simulink model "Context_Diagram"  (R2024a)
settings: Solver=VariableStepAuto  StartTime=0.0  StopTime=10.0  RelTol=1e-3
settings Model: Creator=kmara  LastModifiedBy=chico

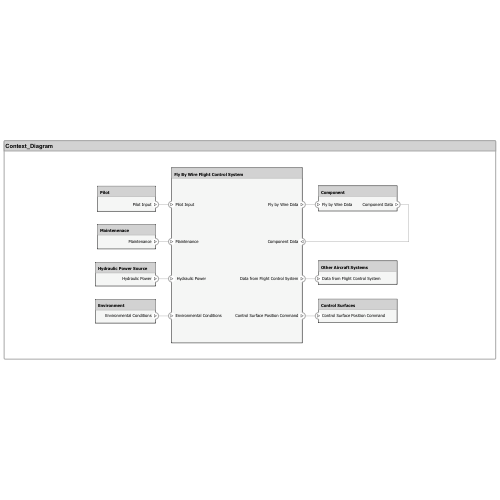
[thumbnail: Simulink's stored preview of the top-level diagram]
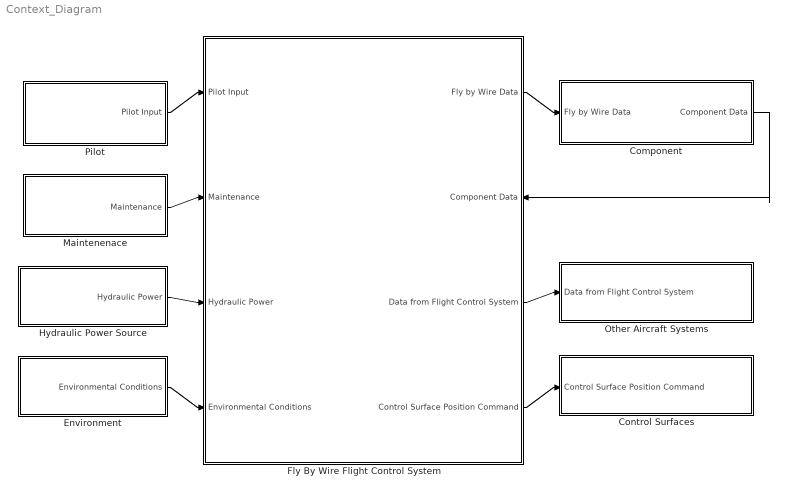
== system Context_Diagram ==
  Component : Subsystem
      settings: PortSchema="{\"entries\":[{\"content\":{\"headerSize\":26,\"margin\":15,\"minimumSpacing\":25,\"sides\":[{\"content\":{\"connectorIds\":[\"In1\"]},\"type\":\"ConnectorPlacement.EquallySpacedRectSide\",\"uuid\":\"b623a921-0a01-4933-aa95-d281e4fd472d\"},{\"content\":{\"connectorIds\":[\"Out1\"],\"side\":\"RIGHT\"},\"type\":\"ConnectorPlacement.EquallySpacedRectSide\",\"uuid\":\"7949cc00-59a5-498d-8900-6268840cf223\"},{\"content\":{\"side\":\"TOP\"},\"type\":\"ConnectorPlacement.EquallySpacedRectSide\",\"uuid\":\"61a6df68-b8b8-47cf-a694-eae6da7c16c5\"}]},\"type\":\"ConnectorPlacement.EquallySpacedConnector\",\"uuid\":\"95d0e082-c8fd-4f2c-a7f4-dd74223482be\"}],\"packageUris\":[\"http://schema.mathworks.com/mf0/Connector/R2020b\"],\"version\":\"1.0\"}"
  Control Surfaces : Subsystem
      settings: PortSchema="{\"entries\":[{\"content\":{\"headerSize\":26,\"margin\":15,\"minimumSpacing\":25,\"sides\":[{\"content\":{\"connectorIds\":[\"In1\"]},\"type\":\"ConnectorPlacement.EquallySpacedRectSide\",\"uuid\":\"b623a921-0a01-4933-aa95-d281e4fd472d\"},{\"content\":{\"side\":\"RIGHT\"},\"type\":\"ConnectorPlacement.EquallySpacedRectSide\",\"uuid\":\"7949cc00-59a5-498d-8900-6268840cf223\"},{\"content\":{\"side\":\"TOP\"},\"type\":\"ConnectorPlacement.EquallySpacedRectSide\",\"uuid\":\"61a6df68-b8b8-47cf-a694-eae6da7c16c5\"}]},\"type\":\"ConnectorPlacement.EquallySpacedConnector\",\"uuid\":\"95d0e082-c8fd-4f2c-a7f4-dd74223482be\"}],\"packageUris\":[\"http://schema.mathworks.com/mf0/Connector/R2020b\"],\"version\":\"1.0\"}"
  Environment : Subsystem
      settings: PortSchema="{\"entries\":[{\"content\":{\"headerSize\":26,\"margin\":15,\"minimumSpacing\":25,\"sides\":[{\"content\":{},\"type\":\"ConnectorPlacement.EquallySpacedRectSide\",\"uuid\":\"b623a921-0a01-4933-aa95-d281e4fd472d\"},{\"content\":{\"connectorIds\":[\"Out1\"],\"side\":\"RIGHT\"},\"type\":\"ConnectorPlacement.EquallySpacedRectSide\",\"uuid\":\"7949cc00-59a5-498d-8900-6268840cf223\"},{\"content\":{\"side\":\"TOP\"},\"type\":\"ConnectorPlacement.EquallySpacedRectSide\",\"uuid\":\"61a6df68-b8b8-47cf-a694-eae6da7c16c5\"}]},\"type\":\"ConnectorPlacement.EquallySpacedConnector\",\"uuid\":\"95d0e082-c8fd-4f2c-a7f4-dd74223482be\"}],\"packageUris\":[\"http://schema.mathworks.com/mf0/Connector/R2020b\"],\"version\":\"1.0\"}"
  Fly By Wire Flight Control System : Subsystem
      settings: PortSchema="{\"entries\":[{\"content\":{\"headerSize\":26,\"margin\":15,\"minimumSpacing\":25,\"sides\":[{\"content\":{\"connectorIds\":[\"In1\",\"In3\",\"In4\",\"In5\"]},\"type\":\"ConnectorPlacement.EquallySpacedRectSide\",\"uuid\":\"b623a921-0a01-4933-aa95-d281e4fd472d\"},{\"content\":{\"connectorIds\":[\"Out2\",\"In2\",\"Out3\",\"Out1\"],\"side\":\"RIGHT\"},\"type\":\"ConnectorPlacement.EquallySpacedRectSide\",\"uuid\":\"7949cc00-59a5-498d-8900-6268840cf223\"},{\"content\":{\"side\":\"TOP\"},\"type\":\"ConnectorPlacement.EquallySpacedRectSide\",\"uuid\":\"61a6df68-b8b8-47cf-a694-eae6da7c16c5\"},{\"content\":{\"side\":\"BOTTOM\"},\"type\":\"ConnectorPlacement.EquallySpacedRectSide\",\"uuid\":\"f40574cc-0ca3-4bc3-ab6d-f0e66dfabfc3\"}]},\"type\":\"ConnectorPlacement.EquallySpacedConnector\",\"uuid\":\"95d0e082-c8fd-4f2c-a7f4-dd74223482be\"}],\"packageUris\":[\"http://schema.mathworks.com/mf0/Connector/R2020b\"],\"version\":\"1.0\"}"
  Hydraulic Power Source : Subsystem
      settings: PortSchema="{\"entries\":[{\"content\":{\"headerSize\":26,\"margin\":15,\"minimumSpacing\":25,\"sides\":[{\"content\":{},\"type\":\"ConnectorPlacement.EquallySpacedRectSide\",\"uuid\":\"b623a921-0a01-4933-aa95-d281e4fd472d\"},{\"content\":{\"connectorIds\":[\"Out1\"],\"side\":\"RIGHT\"},\"type\":\"ConnectorPlacement.EquallySpacedRectSide\",\"uuid\":\"7949cc00-59a5-498d-8900-6268840cf223\"},{\"content\":{\"side\":\"TOP\"},\"type\":\"ConnectorPlacement.EquallySpacedRectSide\",\"uuid\":\"61a6df68-b8b8-47cf-a694-eae6da7c16c5\"}]},\"type\":\"ConnectorPlacement.EquallySpacedConnector\",\"uuid\":\"95d0e082-c8fd-4f2c-a7f4-dd74223482be\"}],\"packageUris\":[\"http://schema.mathworks.com/mf0/Connector/R2020b\"],\"version\":\"1.0\"}"
  Maintenenace : Subsystem
      settings: PortSchema="{\"entries\":[{\"content\":{\"headerSize\":26,\"margin\":15,\"minimumSpacing\":25,\"sides\":[{\"content\":{},\"type\":\"ConnectorPlacement.EquallySpacedRectSide\",\"uuid\":\"b623a921-0a01-4933-aa95-d281e4fd472d\"},{\"content\":{\"connectorIds\":[\"Out1\"],\"side\":\"RIGHT\"},\"type\":\"ConnectorPlacement.EquallySpacedRectSide\",\"uuid\":\"7949cc00-59a5-498d-8900-6268840cf223\"},{\"content\":{\"side\":\"TOP\"},\"type\":\"ConnectorPlacement.EquallySpacedRectSide\",\"uuid\":\"61a6df68-b8b8-47cf-a694-eae6da7c16c5\"}]},\"type\":\"ConnectorPlacement.EquallySpacedConnector\",\"uuid\":\"95d0e082-c8fd-4f2c-a7f4-dd74223482be\"}],\"packageUris\":[\"http://schema.mathworks.com/mf0/Connector/R2020b\"],\"version\":\"1.0\"}"
  Other Aircraft Systems : Subsystem
      settings: PortSchema="{\"entries\":[{\"content\":{\"headerSize\":26,\"margin\":15,\"minimumSpacing\":25,\"sides\":[{\"content\":{\"connectorIds\":[\"In1\"]},\"type\":\"ConnectorPlacement.EquallySpacedRectSide\",\"uuid\":\"b623a921-0a01-4933-aa95-d281e4fd472d\"},{\"content\":{\"side\":\"RIGHT\"},\"type\":\"ConnectorPlacement.EquallySpacedRectSide\",\"uuid\":\"7949cc00-59a5-498d-8900-6268840cf223\"},{\"content\":{\"side\":\"TOP\"},\"type\":\"ConnectorPlacement.EquallySpacedRectSide\",\"uuid\":\"61a6df68-b8b8-47cf-a694-eae6da7c16c5\"}]},\"type\":\"ConnectorPlacement.EquallySpacedConnector\",\"uuid\":\"95d0e082-c8fd-4f2c-a7f4-dd74223482be\"}],\"packageUris\":[\"http://schema.mathworks.com/mf0/Connector/R2020b\"],\"version\":\"1.0\"}"
  Pilot : Subsystem
      settings: PortSchema="{\"entries\":[{\"content\":{\"headerSize\":26,\"margin\":15,\"minimumSpacing\":25,\"sides\":[{\"content\":{},\"type\":\"ConnectorPlacement.EquallySpacedRectSide\",\"uuid\":\"b623a921-0a01-4933-aa95-d281e4fd472d\"},{\"content\":{\"connectorIds\":[\"Out1\"],\"side\":\"RIGHT\"},\"type\":\"ConnectorPlacement.EquallySpacedRectSide\",\"uuid\":\"7949cc00-59a5-498d-8900-6268840cf223\"},{\"content\":{\"side\":\"TOP\"},\"type\":\"ConnectorPlacement.EquallySpacedRectSide\",\"uuid\":\"61a6df68-b8b8-47cf-a694-eae6da7c16c5\"},{\"content\":{\"side\":\"BOTTOM\"},\"type\":\"ConnectorPlacement.EquallySpacedRectSide\",\"uuid\":\"667e63ef-c26a-4d6c-a61f-037a78fc22ca\"}]},\"type\":\"ConnectorPlacement.EquallySpacedConnector\",\"uuid\":\"95d0e082-c8fd-4f2c-a7f4-dd74223482be\"}],\"packageUris\":[\"http://schema.mathworks.com/mf0/Connector/R2020b\"],\"version\":\"1.0\"}"
  wires:
  Pilot/1(Pilot Input) -> Fly By Wire Flight Control System/1(Pilot Input)
  Hydraulic Power Source/1(" Hydraulic Power") -> Fly By Wire Flight Control System/4(" Hydraulic Power")
  Maintenenace/1(Maintenance) -> Fly By Wire Flight Control System/3(Maintenance)
  Component/1(Component Data) -> Fly By Wire Flight Control System/2(Component Data)
  Environment/1(Environmental Conditions) -> Fly By Wire Flight Control System/5(Environmental Conditions)
  Fly By Wire Flight Control System/1(Control Surface Position Command) -> Control Surfaces/1(Control Surface Position Command)
  Fly By Wire Flight Control System/3(Data from Flight Control System) -> Other Aircraft Systems/1(Data from Flight Control System)
  Fly By Wire Flight Control System/2(Fly by Wire Data) -> Component/1(Fly by Wire Data)

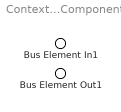
== system Context_Diagram/Component ==
  Bus Element In1 : Inport  PortName=Fly by Wire Data
  Bus Element Out1 : Outport  PortName=Component Data

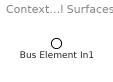
== system Context_Diagram/Control Surfaces ==
  Bus Element In1 : Inport  PortName=Control Surface Position Command

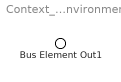
== system Context_Diagram/Environment ==
  Bus Element Out1 : Outport  PortName=Environmental Conditions

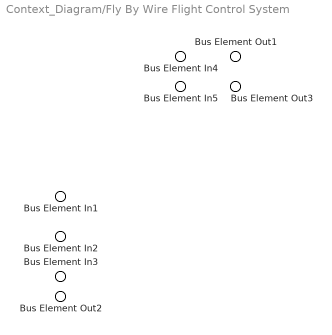
== system Context_Diagram/Fly By Wire Flight Control System ==
  Bus Element In4 : Inport  PortName=Pilot Input
  Bus Element In5 : Inport  Port=2  PortName=Component Data
  Bus Element In1 : Inport  Port=3  PortName=Maintenance
  Bus Element In2 : Inport  Port=4  PortName=Hydraulic Power
  Bus Element In3 : Inport  Port=5  PortName=Environmental Conditions
  Bus Element Out3 : Outport  PortName=Control Surface Position Command
  Bus Element Out1 : Outport  Port=2  PortName=Fly by Wire Data
  Bus Element Out2 : Outport  Port=3  PortName=Data from Flight Control System

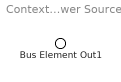
== system Context_Diagram/Hydraulic Power Source ==
  Bus Element Out1 : Outport  PortName=Hydraulic Power

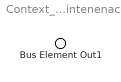
== system Context_Diagram/Maintenenace ==
  Bus Element Out1 : Outport  PortName=Maintenance

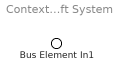
== system Context_Diagram/Other Aircraft Systems ==
  Bus Element In1 : Inport  PortName=Data from Flight Control System

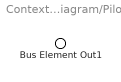
== system Context_Diagram/Pilot ==
  Bus Element Out1 : Outport  PortName=Pilot Input
